simulink model "ActDischarge"  (R2022b)
settings: Solver=FixedStepDiscrete  StartTime=0.0  StopTime=10.0  FixedStep=0.002  RelTol=1e-3
values from neighbouring files (symbols this model uses):
  C_ActDischarge_DischgTim_u16 = 0.0    [ActDisCharge_Sldd.sldd]    (also in ActDisCharge_Sldd_objects.m = myPackage.Parameter)
undefined symbols (not defined in the file or in its folder): ANALOG, ParamCfg_CommandSource_u16, VEHICLE
libraries: simulink x9
settings Model: DataDictionary=ActDisCharge_Sldd.sldd  Creator=ZYH  LastModifiedBy=ZYH
settings OptimizationCC: DefaultParameterBehavior=Inlined  EnhancedBackFolding=on  PassReuseOutputArgsAs=Individual arguments  ZeroInternalMemoryAtStartup=off  OptimizeBlockOrder=speed  DifferentSizesBufferReuse=on  OptimizationCustomize=off  EfficientTunableParamExpr=on
settings DebuggingCC: ParameterTunabilityLossMsg=error
settings SFSimCC: MATLABDynamicMemAlloc=off
settings RTWCC: Description=Embedded Coder  SystemTargetFile=ert.tlc  GenCodeOnly=on  TemplateMakefile=ert_default_tmf
settings CodeAppCC: ForceParamTrailComments=on  IgnoreCustomStorageClasses=off  OperatorAnnotations=on  SimulinkDataObjDesc=on  SFDataObjDesc=on  InsertBlockDesc=on
settings ERTTargetCC: TargetLangStandard=C99 (ISO)  GenerateSampleERTMain=on  InlinedParameterPlacement=NonHierarchical  ERTCustomFileTemplate=example_file_process.tlc

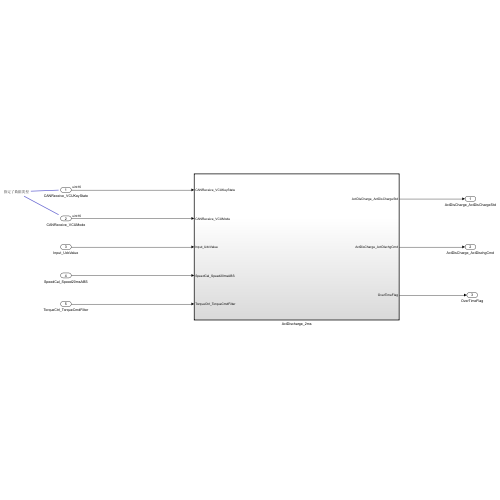
[thumbnail: Simulink's stored preview of the top-level diagram]
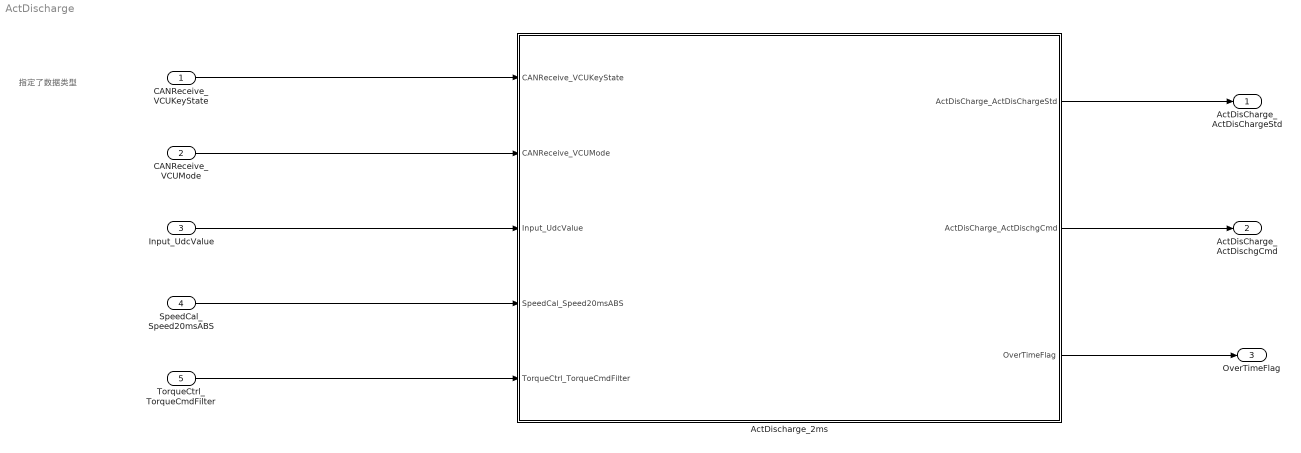
== system ActDischarge ==
  note: 指定了数据类型
  CANReceive_VCUKeyState : Inport  OutDataTypeStr=uint16
  CANReceive_VCUMode : Inport  Port=2  OutDataTypeStr=uint16
  Input_UdcValue : Inport  Port=3
  SpeedCal_Speed20msABS : Inport  Port=4
  TorqueCtrl_TorqueCmdFilter : Inport  Port=5
  ActDischarge_2ms : Subsystem  TreatAsAtomicUnit=on
      settings: RTWSystemCode=Nonreusable function
  ActDisCharge_ActDisChargeStd : Outport
  ActDisCharge_ActDischgCmd : Outport  Port=2
  OverTimeFlag : Outport  Port=3
  wires:
  ActDischarge_2ms/1(ActDisCharge_ActDisChargeStd) -> ActDisCharge_ActDisChargeStd/1
  Input_UdcValue/1 -> ActDischarge_2ms/3(Input_UdcValue)
  SpeedCal_Speed20msABS/1 -> ActDischarge_2ms/4(SpeedCal_Speed20msABS)
  CANReceive_VCUKeyState/1 -> ActDischarge_2ms/1(CANReceive_VCUKeyState)
  CANReceive_VCUMode/1 -> ActDischarge_2ms/2(CANReceive_VCUMode)
  TorqueCtrl_TorqueCmdFilter/1 -> ActDischarge_2ms/5(TorqueCtrl_TorqueCmdFilter)
  ActDischarge_2ms/2(ActDisCharge_ActDischgCmd) -> ActDisCharge_ActDischgCmd/1
  ActDischarge_2ms/3(OverTimeFlag) -> OverTimeFlag/1

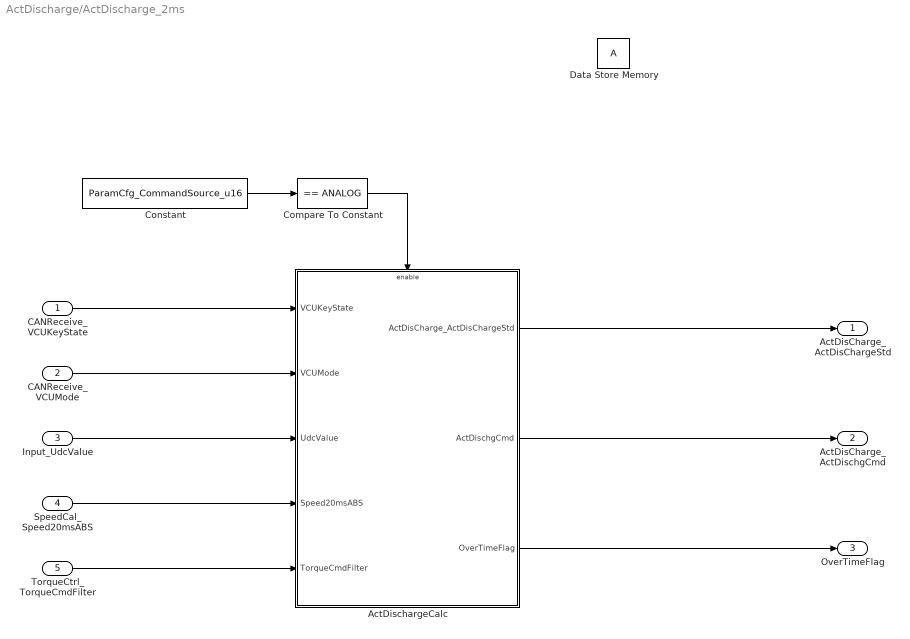
== system ActDischarge/ActDischarge_2ms ==
  CANReceive_VCUKeyState : Inport
  CANReceive_VCUMode : Inport  Port=2
  Input_UdcValue : Inport  Port=3
  SpeedCal_Speed20msABS : Inport  Port=4
  TorqueCtrl_TorqueCmdFilter : Inport  Port=5
  ActDischargeCalc : Subsystem
  Compare To Constant : simulink/Logic and Bit Operations/Compare To Constant  relop===  const=ANALOG  OutDataTypeStr=boolean
  Constant : Constant  Value=ParamCfg_CommandSource_u16
  Data Store Memory : DataStoreMemory  WriteAfterWriteMsg=warning  ShowAdditionalParam=off
  ActDisCharge_ActDisChargeStd : Outport
  ActDisCharge_ActDischgCmd : Outport  Port=2
  OverTimeFlag : Outport  Port=3
  wires:
  CANReceive_VCUKeyState/1 -> ActDischargeCalc/1(VCUKeyState)
  SpeedCal_Speed20msABS/1 -> ActDischargeCalc/4(Speed20msABS)
  Input_UdcValue/1 -> ActDischargeCalc/3(UdcValue)
  CANReceive_VCUMode/1 -> ActDischargeCalc/2(VCUMode)
  TorqueCtrl_TorqueCmdFilter/1 -> ActDischargeCalc/5(TorqueCmdFilter)
  ActDischargeCalc/1(ActDisCharge_ActDisChargeStd) -> ActDisCharge_ActDisChargeStd/1
  Compare To Constant/1 -> ActDischargeCalc/Enable
  Constant/1 -> Compare To Constant/1
  ActDischargeCalc/2(ActDischgCmd) -> ActDisCharge_ActDischgCmd/1
  ActDischargeCalc/3(OverTimeFlag) -> OverTimeFlag/1

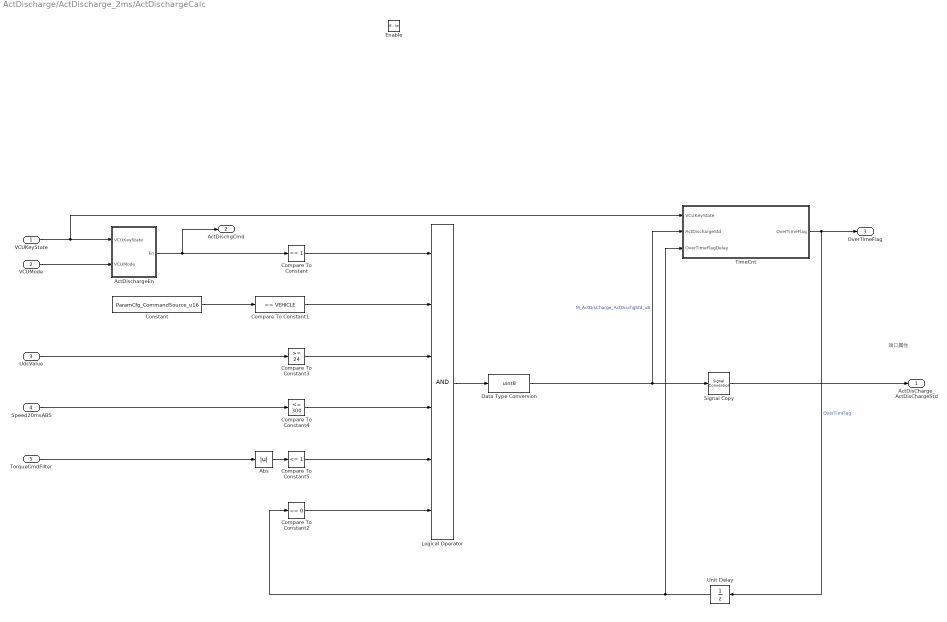
== system ActDischarge/ActDischarge_2ms/ActDischargeCalc ==
  note: 端口属性
  VCUKeyState : Inport
  VCUMode : Inport  Port=2
  UdcValue : Inport  Port=3
  Speed20msABS : Inport  Port=4
  TorqueCmdFilter : Inport  Port=5
  Enable : EnablePort
  Abs : Abs  SaturateOnIntegerOverflow=off
  ActDischargeEn : Subsystem
  Compare To Constant : simulink/Logic and Bit Operations/Compare To Constant  relop===  const=1  OutDataTypeStr=boolean
  Compare To Constant1 : simulink/Logic and Bit Operations/Compare To Constant  relop===  const=VEHICLE  OutDataTypeStr=boolean
  Compare To Constant2 : simulink/Logic and Bit Operations/Compare To Constant  relop===  const=0  OutDataTypeStr=boolean
  Compare To Constant3 : simulink/Logic and Bit Operations/Compare To Constant  relop=>=  const=24  OutDataTypeStr=boolean
  Compare To Constant4 : simulink/Logic and Bit Operations/Compare To Constant  relop=<=  const=300  OutDataTypeStr=boolean
  Compare To Constant5 : simulink/Logic and Bit Operations/Compare To Constant  relop=<=  const=1  OutDataTypeStr=boolean
  Constant : Constant  Value=ParamCfg_CommandSource_u16  OutDataTypeStr=uint16
  Data Type Conversion : DataTypeConversion  OutDataTypeStr=uint8  SaturateOnIntegerOverflow=off  RndMeth=Floor
  Logical Operator : Logic  Inputs=6  AllPortsSameDT=off  OutDataTypeStr=boolean
  Signal Copy : SignalConversion  OverrideOpt=off
  TimeCnt : Subsystem
  Unit Delay : UnitDelay  InitialCondition=false  SampleTime=-1  HasFrameUpgradeWarning=on
  ActDisCharge_ActDisChargeStd : Outport  OutputWhenDisabled=reset  InitialOutput=0
  ActDischgCmd : Outport  Port=2
  OverTimeFlag : Outport  Port=3
  wires:
  VCUKeyState/1 -> TimeCnt/1(VCUKeyState), ActDischargeEn/1(VCUKeyState)
  VCUMode/1 -> ActDischargeEn/2(VCUMode)
  ActDischargeEn/1(En) -> ActDischgCmd/1, Compare To Constant/1
  Constant/1 -> Compare To Constant1/1
  TimeCnt/1(OverTimeFlag) -> OverTimeFlag/1, Unit Delay/1  "OverTimFlag"
  Unit Delay/1 -> Compare To Constant2/1, TimeCnt/3(OverTimeFlagDelay)
  UdcValue/1 -> Compare To Constant3/1
  Speed20msABS/1 -> Compare To Constant4/1
  TorqueCmdFilter/1 -> Abs/1
  Abs/1 -> Compare To Constant5/1
  Compare To Constant2/1 -> Logical Operator/6
  Compare To Constant1/1 -> Logical Operator/2
  Compare To Constant/1 -> Logical Operator/1
  Data Type Conversion/1 -> Signal Copy/1, TimeCnt/2(ActDischargeStd)  "M_ActDisCharge_ActDischgStd_u8"
  Compare To Constant3/1 -> Logical Operator/3
  Compare To Constant4/1 -> Logical Operator/4
  Compare To Constant5/1 -> Logical Operator/5
  Logical Operator/1 -> Data Type Conversion/1
  Signal Copy/1 -> ActDisCharge_ActDisChargeStd/1

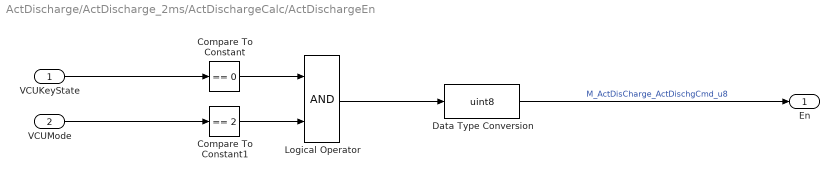
== system ActDischarge/ActDischarge_2ms/ActDischargeCalc/ActDischargeEn ==
  VCUKeyState : Inport
  VCUMode : Inport  Port=2
  Compare To Constant : simulink/Logic and Bit Operations/Compare To Constant  relop===  const=0  OutDataTypeStr=boolean
  Compare To Constant1 : simulink/Logic and Bit Operations/Compare To Constant  relop===  const=2  OutDataTypeStr=boolean
  Data Type Conversion : DataTypeConversion  OutDataTypeStr=uint8  SaturateOnIntegerOverflow=off  RndMeth=Floor
  Logical Operator : Logic  AllPortsSameDT=off  OutDataTypeStr=boolean
  En : Outport
  wires:
  VCUKeyState/1 -> Compare To Constant/1
  VCUMode/1 -> Compare To Constant1/1
  Compare To Constant1/1 -> Logical Operator/2
  Compare To Constant/1 -> Logical Operator/1
  Data Type Conversion/1 -> En/1  "M_ActDisCharge_ActDischgCmd_u8"
  Logical Operator/1 -> Data Type Conversion/1

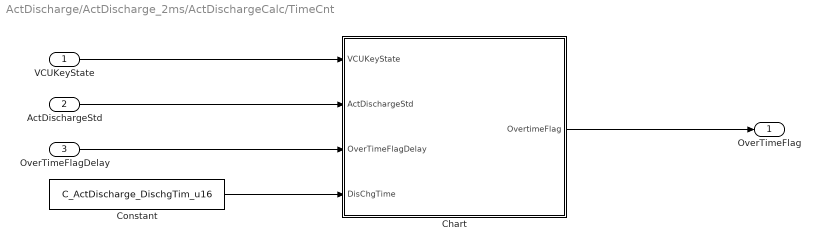
== system ActDischarge/ActDischarge_2ms/ActDischargeCalc/TimeCnt ==
  VCUKeyState : Inport
  ActDischargeStd : Inport  Port=2
  OverTimeFlagDelay : Inport  Port=3
  Chart : Stateflow chart  TreatAsAtomicUnit=on
  Constant : Constant  Value=C_ActDischarge_DischgTim_u16
  OverTimeFlag : Outport
  wires:
  ActDischargeStd/1 -> Chart/2(ActDischargeStd)
  VCUKeyState/1 -> Chart/1(VCUKeyState)
  OverTimeFlagDelay/1 -> Chart/3(OverTimeFlagDelay)
  Constant/1 -> Chart/4(DisChgTime)
  Chart/1(OvertimeFlag) -> OverTimeFlag/1

== stateflow chart ActDischarge/ActDischarge_2ms/ActDischargeCalc/TimeCnt/Chart ==
  (default) -> (junction 4)
  (junction 4) -> (junction 6) [order 1] : [ActDischargeStd == true && OverTimeFlagDelay == false]
  (junction 4) -> (junction 21) [order 2]
  (junction 6) -> (junction 9)
  (junction 9) -> (junction 11) [order 1] : [TimeCnt > DisChgTime ]
  (junction 9) -> (junction 18) [order 2] : {TimeCnt = TimeCnt +1}
  (junction 11) -> (junction 14) : {
      | TimeCnt = DisChgTime
      | OvertimeFlag = true
      | }
  (junction 14) -> (junction 18)
  (junction 18) -> (junction 34)
  (junction 21) -> (junction 23) [order 2] : [VCUKeyState == 1]
  (junction 21) -> (junction 27) [order 1]
  (junction 23) -> (junction 43) : {
      | OvertimeFlag = false
      | TimeCnt = 0
      | }
  (junction 43) -> (junction 27)
  (junction 27) -> (junction 30)
  (junction 34) -> (junction 30)
  (junction 30) -> (junction 37)
  data: VCUKeyState input; ActDischargeStd input; OverTimeFlagDelay input; DisChgTime input; TimeCnt local uint16 =0; OvertimeFlag output uint8 =0
